simulink model "tanque"  (R2022b)
settings: Solver=VariableStepAuto  StartTime=0.0  StopTime=10.0  RelTol=1e-3
undefined symbols (not defined in the file or in its folder): a, A, b
settings Model: Creator=emmanuel  LastModifiedBy=emmanuel

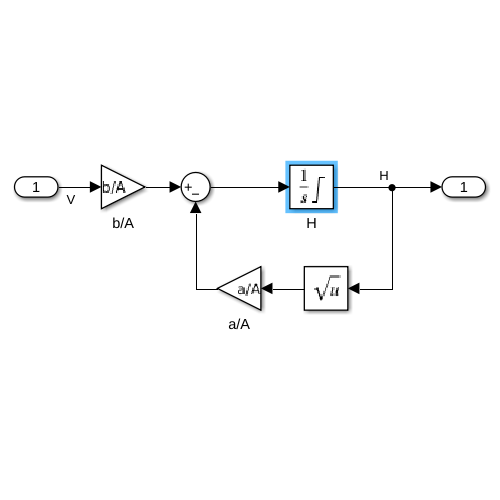
[thumbnail: Simulink's stored preview of the top-level diagram]
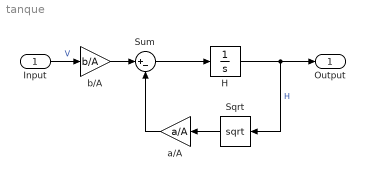
== system tanque ==
  Input : Inport
  H : Integrator  InitialCondition=0.2  LimitOutput=on  UpperSaturationLimit=0.62  LowerSaturationLimit=0
  Sqrt : Sqrt
  Sum : Sum  Inputs=|+-  SaturateOnIntegerOverflow=on
  a/A : Gain  Gain=a/A  SaturateOnIntegerOverflow=on  OutDataTypeStr=Inherit: Same as input  ParamDataTypeStr=Inherit: Same as input
  b/A : Gain  Gain=b/A  SaturateOnIntegerOverflow=on  OutDataTypeStr=Inherit: Same as input  ParamDataTypeStr=Inherit: Same as input
  Output : Outport  VectorParamsAs1DForOutWhenUnconnected=off
  wires:
  Sum/1 -> H/1
  H/1 -> Sqrt/1, Output/1  "H"
  Input/1 -> b/A/1  "V"
  Sqrt/1 -> a/A/1
  b/A/1 -> Sum/1
  a/A/1 -> Sum/2
